simulink model "Sistema3"  (R2017b)
settings: Solver=VariableStepAuto  StartTime=0.0  StopTime=10.0  RelTol=1e-3
values from neighbouring files (symbols this model uses):
  Cs = tf(Crl)    [main.m]
  Fs = tf(Frl)    [main.m]
  Gs = tf([112], [1 4.06 11.98 23.9])    [main.m]
libraries: simulink x1
settings Model: Creator=felip  LastModifiedBy=felip

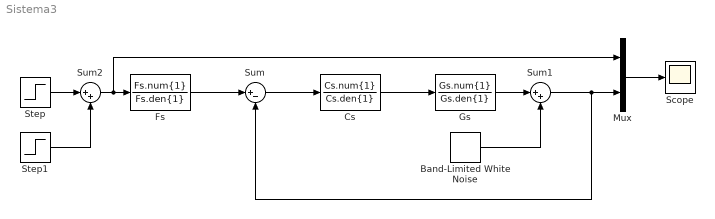
== system Sistema3 ==
  Band-Limited White Noise : simulink/Sources/Band-Limited White Noise  Cov=[0.000001]  Ts=0.01  seed=[23341]
  Cs : TransferFcn  Numerator=Cs.num{1}  Denominator=Cs.den{1}
  Fs : TransferFcn  Numerator=Fs.num{1}  Denominator=Fs.den{1}
  Gs : TransferFcn  Numerator=Gs.num{1}  Denominator=Gs.den{1}
  Mux : Mux  Inputs=2
  Scope : Scope
  Step : Step  SampleTime=0
  Step1 : Step  Time=2  SampleTime=0
  Sum : Sum  Inputs=|+-
  Sum1 : Sum  Inputs=|++
  Sum2 : Sum  Inputs=|++
  wires:
  Mux/1 -> Scope/1
  Sum1/1 -> Sum/2, Mux/2
  Cs/1 -> Gs/1
  Sum/1 -> Cs/1
  Fs/1 -> Sum/1
  Sum2/1 -> Mux/1, Fs/1
  Step/1 -> Sum2/1
  Step1/1 -> Sum2/2
  Gs/1 -> Sum1/1
  Band-Limited White Noise/1 -> Sum1/2
